simulink model "MRACDiretoTrab1AutoCriterio2"  (R2015a)
settings: Solver=ode45  StartTime=0.0  StopTime=360000  RelTol=1e-3
undefined symbols (not defined in the file): b, gamma, it, ref, theta_c_ini
libraries: simulink x7
settings Model: Creator=user  LastModifiedBy=user

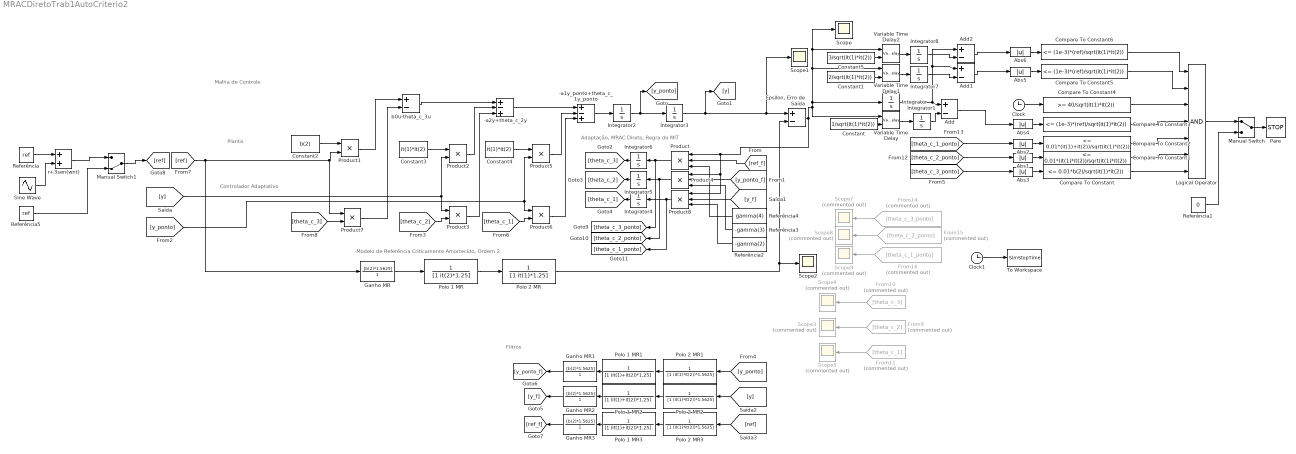
== system MRACDiretoTrab1AutoCriterio2 ==
  note: Filtros
  note: Planta
  note: Malha de Controle
  note: Modelo de Referência Criticamente Amortecido, Ordem 2
  note: Controlador Adaptativo
  note: Adaptação, MRAC Direto, Regra do MIT
  "  Referência" : Constant  Value=ref
  "  Referência1" : Constant  Value=0
  "  Referência2" : Constant  Value=-gamma(2)
  "  Referência3" : Constant  Value=-gamma(3)
  "  Referência4" : Constant  Value=gamma(4)
  "  Referência5" : Constant  Value=ref
  -a1y_ponto+theta_c_1y_ponto : Sum  Inputs=+-+
  -a2y+theta_c_2y : Sum  Inputs=+-+
  Abs{1..6} (6 alike) : Abs
  Add : Sum  Inputs=+-
  Add1 : Sum  Inputs=+-
  Add2 : Sum  Inputs=+-
  Clock : Clock
  Clock1 : Clock
  Compare To Constant : simulink/Logic and Bit Operations/Compare To Constant  relop=<=  const=0.01*b(2)/sqrt(it(1)*it(2))  OutDataTypeStr=boolean
  Compare To Constant1 : simulink/Logic and Bit Operations/Compare To Constant  relop=<=  const=0.01*(it(1)*it(2))/sqrt(it(1)*it(2))  OutDataTypeStr=boolean
  Compare To Constant2 : simulink/Logic and Bit Operations/Compare To Constant  relop=<=  const=0.01*(it(1)+it(2))/sqrt(it(1)*it(2))  OutDataTypeStr=boolean
  Compare To Constant3 : simulink/Logic and Bit Operations/Compare To Constant  relop=<=  const=(1e-3)*(ref)/sqrt(it(1)*it(2))  OutDataTypeStr=boolean
  Compare To Constant4 : simulink/Logic and Bit Operations/Compare To Constant  relop=>=  const=40/sqrt(it(1)*it(2))  OutDataTypeStr=boolean
  Compare To Constant5 : simulink/Logic and Bit Operations/Compare To Constant  relop=<=  const=(1e-3)*(ref)/sqrt(it(1)*it(2))  OutDataTypeStr=boolean
  Compare To Constant6 : simulink/Logic and Bit Operations/Compare To Constant  relop=<=  const=(1e-3)*(ref)/sqrt(it(1)*it(2))  OutDataTypeStr=boolean
  Constant : Constant  Value=1/sqrt(it(1)*it(2))
  Constant1 : Constant  Value=2/sqrt(it(1)*it(2))
  Constant2 : Constant  Value=b(2)
  Constant3 : Constant  Value=it(1)*it(2)
  Constant4 : Constant  Value=it(1)*it(2)
  Constant5 : Constant  Value=3/sqrt(it(1)*it(2))
  "Epsilon, Erro de Saída" : Sum  Inputs=+-
  From10 : From  Commented=on  GotoTag=theta_c_3
  From11 : From  Commented=on  GotoTag=theta_c_1
  From14 : From  Commented=on  GotoTag=theta_c_3_ponto
  From15 : From  Commented=on  GotoTag=theta_c_2_ponto
  From16 : From  Commented=on  GotoTag=theta_c_1_ponto
  From9 : From  Commented=on  GotoTag=theta_c_2
  Ganho MR{,1..3} (4 alike) : TransferFcn  Numerator=[b(2)*1.5625]  Denominator=[1]
  Integrator{,1..3,7..8} (6 alike) : Integrator
  Integrator4 : Integrator  InitialCondition=theta_c_ini(4)
  Integrator5 : Integrator  InitialCondition=theta_c_ini(3)
  Integrator6 : Integrator  InitialCondition=theta_c_ini(2)
  Logical Operator : Logic  Inputs=7  AllPortsSameDT=off  OutDataTypeStr=boolean
  Manual Switch : ManualSwitch
  Manual Switch1 : ManualSwitch  CurrentSetting=0
  Pare : Stop
  Polo 1 MR : TransferFcn  Denominator=[1 it(2)*1.25]
  Polo 1 MR1 : TransferFcn  Denominator=[1 (it(1)+it(2))*1.25]
  Polo 1 MR2 : TransferFcn  Denominator=[1 (it(1)+it(2))*1.25]
  Polo 1 MR3 : TransferFcn  Denominator=[1 (it(1)+it(2))*1.25]
  Polo 2 MR : TransferFcn  Denominator=[1 it(1)*1.25]
  Polo 2 MR1 : TransferFcn  Denominator=[1 (it(1)*it(2))*1.5625]
  Polo 2 MR2 : TransferFcn  Denominator=[1 (it(1)*it(2))*1.5625]
  Polo 2 MR3 : TransferFcn  Denominator=[1 (it(1)*it(2))*1.5625]
  Product : Product  Inputs=3
  Product{1..3,5..7} (6 alike) : Product
  Product4 : Product  Inputs=3
  Product8 : Product  Inputs=3
  Scope : Scope
      settings: YMin=4.06502e-07  YMax=4.06508e-07
  Scope1 : Scope
      settings: YMin=-100  YMax=125
  Scope2 : Scope
      settings: YMin=100  YMax=100  SaveName=ScopeData2
  Scope{3..5,7..9} (6 alike) : Scope  Commented=on
      Scope3 settings: YMin=1.92512  YMax=1.92512  SaveName=ScopeData3
      Scope4 settings: YMin=3.045  YMax=3.0725  SaveName=ScopeData4
      Scope5 settings: YMin=9.39  YMax=9.48  SaveName=ScopeData5
      Scope7 settings: YMin=-1.095e-05  YMax=-1.045e-05  SaveName=ScopeData7
      Scope8 settings: YMin=95  YMax=105  SaveName=ScopeData8
      Scope9 settings: YMin=95  YMax=105  SaveName=ScopeData9
  Sine Wave : Sin  Amplitude=ref/4  Frequency=sqrt(it(1)*it(2)*1.5625)  SampleTime=0
  To Workspace : ToWorkspace  VariableName=SimStopTime  SaveFormat=Timeseries  SampleTime=-1
  Variable Time Delay : VariableTransportDelay  MaximumDelay=10
  Variable Time Delay1 : VariableTransportDelay  MaximumDelay=10
  Variable Time Delay2 : VariableTransportDelay  MaximumDelay=10
  b0u-theta_c_3u : Sum  Inputs=+-
  r+3sen(wnt) : Sum
  wires:
  Ganho MR/1 -> Polo 1 MR/1
  Polo 1 MR/1 -> Polo 2 MR/1
  Polo 2 MR/1 -> Scope2/1, "Epsilon, Erro de Saída"/2
  Integrator3/1 -> [y], Scope1/1, "Epsilon, Erro de Saída"/1
  Integrator2/1 -> [y_ponto], Integrator3/1
  -a1y_ponto+theta_c_1y_ponto/1 -> Integrator2/1
  -a2y+theta_c_2y/1 -> -a1y_ponto+theta_c_1y_ponto/1
  Product2/1 -> -a2y+theta_c_2y/2
  Constant3/1 -> Product2/1
  b0u-theta_c_3u/1 -> -a2y+theta_c_2y/1
  [y] -> Product2/2, Product3/1
  Product3/1 -> -a2y+theta_c_2y/3
  [theta_c_2] -> Product3/2
  Constant4/1 -> Product5/1
  [y_ponto] -> Product6/1, Product5/2
  [theta_c_1] -> Product6/2
  Product5/1 -> -a1y_ponto+theta_c_1y_ponto/2
  Product6/1 -> -a1y_ponto+theta_c_1y_ponto/3
  Constant2/1 -> Product1/1
  [theta_c_3] -> Product7/2
  Product1/1 -> b0u-theta_c_3u/1
  Product7/1 -> b0u-theta_c_3u/2
  [ref_f] -> Product/2
  [y_ponto_f] -> Product4/2
  [y_f] -> Product8/2
  "  Referência4"/1 -> Product/3
  "  Referência3"/1 -> Product4/3
  "  Referência2"/1 -> Product8/3
  Polo 2 MR1/1 -> Polo 1 MR1/1
  Polo 1 MR1/1 -> Ganho MR1/1
  [y_ponto] -> Polo 2 MR1/1
  Polo 2 MR2/1 -> Polo 1 MR2/1
  Polo 1 MR2/1 -> Ganho MR2/1
  [y] -> Polo 2 MR2/1
  Ganho MR1/1 -> [y_ponto_f]
  Ganho MR2/1 -> [y_f]
  Polo 2 MR3/1 -> Polo 1 MR3/1
  Polo 1 MR3/1 -> Ganho MR3/1
  [ref] -> Polo 2 MR3/1
  Ganho MR3/1 -> [ref_f]
  Integrator4/1 -> [theta_c_1]
  Product/1 -> [theta_c_3_ponto], Integrator6/1
  Integrator6/1 -> [theta_c_3]
  Product4/1 -> [theta_c_2_ponto], Integrator5/1
  Integrator5/1 -> [theta_c_2]
  [ref] -> Ganho MR/1, Product7/1, Product1/2
  "  Referência"/1 -> r+3sen(wnt)/1
  Sine Wave/1 -> r+3sen(wnt)/2
  From9/1 -> Scope3/1
  From10/1 -> Scope4/1
  From11/1 -> Scope5/1
  Product8/1 -> [theta_c_1_ponto], Integrator4/1
  Compare To Constant/1 -> Logical Operator/7
  Compare To Constant1/1 -> Logical Operator/6
  Compare To Constant2/1 -> Logical Operator/5
  "Epsilon, Erro de Saída"/1 -> Variable Time Delay1/1, Variable Time Delay2/1, Scope/1, Integrator/1, Variable Time Delay/1, Product8/1, Product4/1, Product/1
  Compare To Constant3/1 -> Logical Operator/4
  Clock/1 -> Compare To Constant4/1
  Compare To Constant4/1 -> Logical Operator/3
  Abs3/1 -> Compare To Constant/1
  Abs1/1 -> Compare To Constant1/1
  [theta_c_3_ponto] -> Abs3/1
  [theta_c_2_ponto] -> Abs1/1
  [theta_c_1_ponto] -> Abs2/1
  Abs4/1 -> Compare To Constant3/1
  Abs2/1 -> Compare To Constant2/1
  Variable Time Delay/1 -> Integrator1/1
  Integrator/1 -> Add1/1, Add2/1, Add/1
  Integrator1/1 -> Add/2
  Constant/1 -> Variable Time Delay/2
  Add/1 -> Abs4/1
  From14/1 -> Scope7/1
  From15/1 -> Scope8/1
  From16/1 -> Scope9/1
  Constant1/1 -> Variable Time Delay1/2
  Variable Time Delay1/1 -> Integrator7/1
  Constant5/1 -> Variable Time Delay2/2
  Variable Time Delay2/1 -> Integrator8/1
  Integrator7/1 -> Add1/2
  Integrator8/1 -> Add2/2
  Compare To Constant5/1 -> Logical Operator/2
  Compare To Constant6/1 -> Logical Operator/1
  Logical Operator/1 -> Manual Switch/1
  Manual Switch/1 -> Pare/1
  "  Referência1"/1 -> Manual Switch/2
  Manual Switch1/1 -> [ref]
  r+3sen(wnt)/1 -> Manual Switch1/1
  "  Referência5"/1 -> Manual Switch1/2
  Abs6/1 -> Compare To Constant6/1
  Add2/1 -> Abs6/1
  Add1/1 -> Abs5/1
  Abs5/1 -> Compare To Constant5/1
  Clock1/1 -> To Workspace/1
